simulink model "Motor"  (Simulink 8.8)
settings: Solver=ode45  StartTime=0.0  StopTime=2  RelTol=1e-3  EnableMultiTasking=on
values from neighbouring files (symbols this model uses):
  J = 4*10^-5    (= 4e-05)    [Motor_DATA.m]
  Ki_n = 0.0351    [Motor_DATA.m]
  km = 0.0325    [Motor_DATA.m]
  Kp_n = 0.00048    [Motor_DATA.m]
  RA = 5.8    [Motor_DATA.m]
  TA = LA / RA    (= 0.000129310344828)    [Motor_DATA.m]
  ts_n = 0.015    [Motor_DATA.m]
undefined symbols (not defined in the file or in its folder): sigbuilder_block
libraries: simulink x1
CloseFcn:
  | rtwprivate ssgencode ModelCloseRequest Motor
settings Model: SuppressorTable=22 serialization::archive 11 0 3 0 0 0 0 0  Creator=dfr4286  LastModifiedBy=roman
settings OptimizationCC: DefaultParameterBehavior=Inlined  UseDivisionForNetSlopeComputation=on  UseFloatMulNetSlope=on  InlineInvariantSignals=on  PassReuseOutputArgsAs=Individual arguments  ExpressionDepthLimit=2147483647  ZeroExternalMemoryAtStartup=off  ZeroInternalMemoryAtStartup=off  NoFixptDivByZeroProtection=on  EfficientFloat2IntCast=on  LifeSpan=1
settings DebuggingCC: SolverPrmCheckMsg=warning
settings HardwareCC: ProdBitPerPointer=64  ProdBitPerSizeT=64  ProdBitPerPtrDiffT=64  ProdLargestAtomicFloat=Float  ProdIntDivRoundTo=Zero  ProdEndianess=LittleEndian  ProdWordSize=64  ProdHWDeviceType=Intel->x86-64 (Windows64)
settings RTWCC: SystemTargetFile=ert.tlc  TemplateMakefile=ert_default_tmf  Description=Real-Time Workshop Embedded Coder  GenerateReport=on  IncludeHyperlinkInReport=on  LaunchReport=on  GenerateTraceInfo=on  GenerateTraceReport=on  GenerateTraceReportSl=on  GenerateTraceReportSf=on  GenerateTraceReportEml=on  GenerateCodeMetricsReport=on
settings CodeAppCC: ForceParamTrailComments=on  IgnoreCustomStorageClasses=off  SimulinkDataObjDesc=on  CustomSymbolStrGlobalVar=rt$N$M  CustomSymbolStrType=$N$M  CustomSymbolStrFcn=$N$M$F  CustomSymbolStrMacro=$N$M  InsertBlockDesc=on  InternalIdentifier=Classic
settings ERTTargetCC: MultiwordLength=2048  GenerateSampleERTMain=on  CombineSignalStateStructs=on  SupportComplex=off  InlinedParameterPlacement=NonHierarchical  TargetOS=VxWorksExample  ERTCustomFileTemplate=example_file_process.tlc  ERTFilePackagingFormat=CompactWithDataFile  ConvertIfToSwitch=off  SuppressUnreachableDefaultCases=off

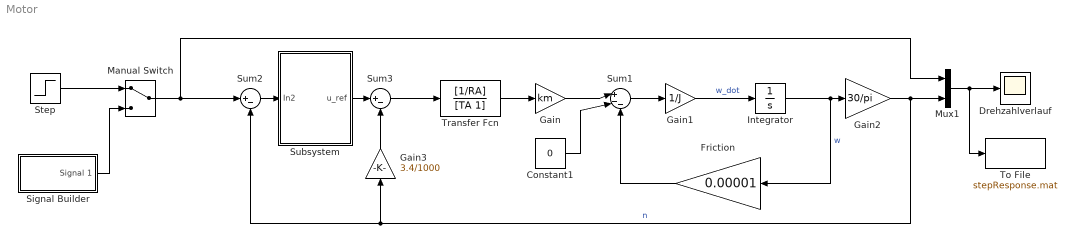
== system Motor ==
  Constant1 : Constant  Value=0
  Drehzahlverlauf : Scope
  Friction : Gain  Gain=0.00001
  Gain : Gain  Gain=km
  Gain1 : Gain  Gain=1/J
  Gain2 : Gain  Gain=30/pi
  Gain3 : Gain  Gain=3.4/1000
  Integrator : Integrator
  Manual Switch : ManualSwitch
  Mux1 : Mux  Inputs=2
  Signal Builder : Subsystem  Tag=STV Subsys  LoadFcn=sigbuilder_block('load');  StartFcn=sigbuilder_block('start');  StopFcn=sigbuilder_block('stop');  ClipboardFcn=sigbuilder_block('clipboard');  mask(Sigbuilder block){tuvar=[0:10]}
      mask help: Sigbuilder GUI
      mask init:
      | if ~strcmp(get_param(bdroot(gcbh),'SimulationStatus'),'stopped') tuvar = sigbuilder_block('maskInit'); end
      settings: CopyFcn=sigbuilder_block('copy');  DeleteFcn=sigbuilder_block('delete');  ModelCloseFcn=sigbuilder_block('modelClose');  PreSaveFcn=sigbuilder_block('preSave');  PauseFcn=sigbuilder_block('pause')  ContinueFcn=sigbuilder_block('continue')  NameChangeFcn=sigbuilder_block('namechange');  OpenFcn=sigbuilder_block('open',[0 4 1680 950 ]);  CloseFcn=sigbuilder_block('close');
      mask Display: plot(0,0,100,100,[10,10,40,40,10],[80,20,20,80,80],[40,10],[50,50], [40,27,10],[65,72,56],[40,25,25,10],[28,28,43,43]);
  Step : Step  Time=0.1  After=1000  SampleTime=0
  Subsystem : Subsystem
  Sum1 : Sum  Inputs=|+--
  Sum2 : Sum  Inputs=|+-
  Sum3 : Sum  Inputs=|+-
  To File : ToFile  Filename=stepResponse.mat
  Transfer Fcn : TransferFcn  Numerator=[1/RA]  Denominator=[TA 1]
  wires:
  Transfer Fcn/1 -> Gain/1
  Gain/1 -> Sum1/1
  Sum1/1 -> Gain1/1
  Gain1/1 -> Integrator/1  "w_dot"
  Integrator/1 -> Friction/1, Gain2/1  "w"
  Gain2/1 -> Sum2/2, Gain3/1, Mux1/2  "n"
  Step/1 -> Manual Switch/1
  Manual Switch/1 -> Sum2/1, Mux1/1
  Sum2/1 -> Subsystem/1(In2)
  Sum3/1 -> Transfer Fcn/1
  Gain3/1 -> Sum3/2
  Friction/1 -> Sum1/3
  Constant1/1 -> Sum1/2
  Signal Builder/1(Signal 1) -> Manual Switch/2
  Mux1/1 -> Drehzahlverlauf/1, To File/1
  Subsystem/1(u_ref) -> Sum3/1

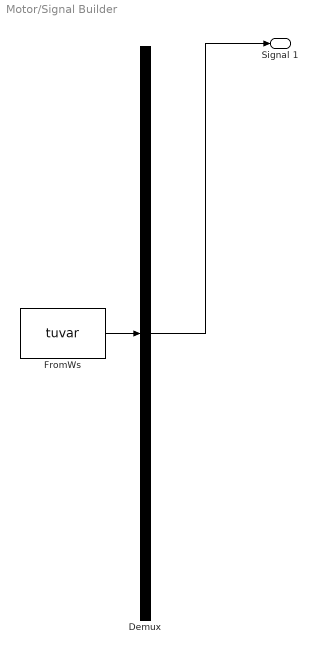
== system Motor/Signal Builder ==
  Demux : Demux  Tag=STV Demux  Outputs=1
  FromWs : FromWorkspace  Tag=STV FromWs  VariableName=tuvar  SampleTime=0  SigBuilderData=DataTag0  VnvData=DataTag1
      SigBuilderData=|
      | common.afterFinalStr = 'Extrapolate'
      | common.sampleTime = 0
      | dataSet.timeRange = [0 10]
      | dataSet.name = 'Group 1'
      | sbobj.Groups.Name = 'Group 1'
      | sbobj.Groups.Signals.Name = 'Signal 1'
      | sbobj.Groups.Signals.XData = [0 5 5 9.9 10]
      | sbobj.Groups.Signals.YData = [1000 1000 -2000 -2000 0]
  Signal 1 : Outport  Tag=STV Outport
  wires:
  Demux/1 -> Signal 1/1
  FromWs/1 -> Demux/1

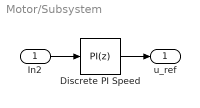
== system Motor/Subsystem ==
  In2 : Inport
  Discrete PI Speed : simulink/Continuous/PID Controller  Controller=PI  TimeDomain=Discrete-time  SampleTime=ts_n  IntegratorMethod=Forward Euler  FilterMethod=Forward Euler  Form=Parallel  UseFilter=on  ControllerParametersSource=internal  P=Kp_n  I=Ki_n  D=0  N=100  InitialConditionSource=internal  InitialConditionForIntegrator=0  InitialConditionForFilter=0  ExternalReset=none  LimitOutput=on  UpperSaturationLimit=18  LowerSaturationLimit=-18  LinearizeAsGain=off  AntiWindupMode=back-calculation  Kb=Ki_n  TrackingMode=off  Kt=1  PParamMin=[]  PParamMax=[]  IParamMin=[]  IParamMax=[]  DParamMin=[]  DParamMax=[]  NParamMin=[]  NParamMax=[]  KbParamMin=[]  KbParamMax=[]  KtParamMin=[]  KtParamMax=[]  POutMin=[]  POutMax=[]  IOutMin=[]  IOutMax=[]  DOutMin=[]  DOutMax=[]  NOutMin=[]  NOutMax=[]  KbOutMin=[]  KbOutMax=[]  KtOutMin=[]  KtOutMax=[]  IntegratorOutMin=[]  IntegratorOutMax=[]  FilterOutMin=[]  FilterOutMax=[]  SumOutMin=[]  SumOutMax=[]  SumI1OutMin=[]  SumI1OutMax=[]  SumI2OutMin=[]  SumI2OutMax=[]  SumI3OutMin=[]  SumI3OutMax=[]  SumDOutMin=[]  SumDOutMax=[]  SaturationOutMin=[]  SaturationOutMax=[]  IntegratorContinuousStateAttributes=''  IntegratorStateMustResolveToSignalObject=off  IntegratorRTWStateStorageClass=Auto  FilterContinuousStateAttributes=''  FilterStateMustResolveToSignalObject=off  FilterRTWStateStorageClass=Auto  DifferentiatorICPrevScaledInput=0  DifferentiatorOutMin=[]  DifferentiatorOutMax=[]
  u_ref : Outport
  wires:
  In2/1 -> Discrete PI Speed/1
  Discrete PI Speed/1 -> u_ref/1
